simulink model "Demo_MinDef_Aug2013"  (Simulink 7.7)
settings: Solver=ode4  StartTime=0.0  StopTime=inf  FixedStep=sample_time_Vicon  RelTol=1e-3
InitFcn:
  | sample_time_Vicon = 0.005;
  | sample_time=0.02;
  | DeltaT = sample_time;
  | H0 = 0.35;
  | Kl = 1;
  | Omega_r =1.2; %1.2
  | Omega_c = 1.2;
  | omega_circle = 36*pi/180;
  | omega_h = 0.1;%Ascending speed
  | PI = pi;
undefined symbols (not defined in the file or in its folder): DiscIntNeverNeededParam
libraries: simulink x22, dspadpt3 x8
(part 4 of 4)

== system Demo_MinDef_Aug2013/Vicon_Data/Raw Quad Pose from Vicon/Process Vicon Raw Data1/Flip_pi1/Flip_0_to_2pi/Flip_2pi ==
  Angle : Inport
  Bias : Bias  Bias=-2*pi
  Constant : Constant  Value=2*pi
  Data Type Duplicate : DataTypeDuplicate
  Modulo : Math  Operator=mod  SaturateOnIntegerOverflow=on
  Sign1 : Signum
  Switch : Switch
  Angle_Flip : Outport
  wires:
  Angle/1 -> Modulo/1, Sign1/1, Data Type Duplicate/1
  Constant/1 -> Modulo/2
  Modulo/1 -> Bias/1, Switch/1
  Sign1/1 -> Switch/2
  Bias/1 -> Switch/3
  Switch/1 -> Angle_Flip/1, Data Type Duplicate/2

== system Demo_MinDef_Aug2013/Vicon_Data/Raw Quad Pose from Vicon/Process Vicon Raw Data2/Flip_pi1/Flip_0_to_2pi/Flip_2pi ==
  Angle : Inport
  Bias : Bias  Bias=-2*pi
  Constant : Constant  Value=2*pi
  Data Type Duplicate : DataTypeDuplicate
  Modulo : Math  Operator=mod  SaturateOnIntegerOverflow=on
  Sign1 : Signum
  Switch : Switch
  Angle_Flip : Outport
  wires:
  Switch/1 -> Data Type Duplicate/2, Angle_Flip/1
  Bias/1 -> Switch/3
  Sign1/1 -> Switch/2
  Modulo/1 -> Switch/1, Bias/1
  Constant/1 -> Modulo/2
  Angle/1 -> Data Type Duplicate/1, Sign1/1, Modulo/1

== system Demo_MinDef_Aug2013/Vicon_Data/Raw Quad Pose from Vicon/Process Vicon Raw Data3/Flip_pi1/Flip_0_to_2pi/Flip_2pi ==
  Angle : Inport
  Bias : Bias  Bias=-2*pi
  Constant : Constant  Value=2*pi
  Data Type Duplicate : DataTypeDuplicate
  Modulo : Math  Operator=mod  SaturateOnIntegerOverflow=on
  Sign1 : Signum
  Switch : Switch
  Angle_Flip : Outport
  wires:
  Angle/1 -> Modulo/1, Sign1/1, Data Type Duplicate/1
  Constant/1 -> Modulo/2
  Modulo/1 -> Bias/1, Switch/1
  Sign1/1 -> Switch/2
  Bias/1 -> Switch/3
  Switch/1 -> Angle_Flip/1, Data Type Duplicate/2

== system Demo_MinDef_Aug2013/Vicon_Data/Raw Quad Pose from Vicon/Process Vicon Raw Data4/Flip_pi1/Flip_0_to_2pi/Flip_2pi ==
  Angle : Inport
  Bias : Bias  Bias=-2*pi
  Constant : Constant  Value=2*pi
  Data Type Duplicate : DataTypeDuplicate
  Modulo : Math  Operator=mod  SaturateOnIntegerOverflow=on
  Sign1 : Signum
  Switch : Switch
  Angle_Flip : Outport
  wires:
  Switch/1 -> Data Type Duplicate/2, Angle_Flip/1
  Bias/1 -> Switch/3
  Sign1/1 -> Switch/2
  Modulo/1 -> Switch/1, Bias/1
  Constant/1 -> Modulo/2
  Angle/1 -> Data Type Duplicate/1, Sign1/1, Modulo/1

== system Demo_MinDef_Aug2013/Vicon_Data/Raw Quad Pose from Vicon/Process Vicon Raw Data5/Flip_pi1/Flip_0_to_2pi/Flip_2pi ==
  Angle : Inport
  Bias : Bias  Bias=-2*pi
  Constant : Constant  Value=2*pi
  Data Type Duplicate : DataTypeDuplicate
  Modulo : Math  Operator=mod  SaturateOnIntegerOverflow=on
  Sign1 : Signum
  Switch : Switch
  Angle_Flip : Outport
  wires:
  Switch/1 -> Data Type Duplicate/2, Angle_Flip/1
  Bias/1 -> Switch/3
  Sign1/1 -> Switch/2
  Modulo/1 -> Switch/1, Bias/1
  Constant/1 -> Modulo/2
  Angle/1 -> Data Type Duplicate/1, Sign1/1, Modulo/1

== system Demo_MinDef_Aug2013/Vicon_Data/Raw Quad Pose from Vicon/Process Vicon Raw Data6/Flip_pi1/Flip_0_to_2pi/Flip_2pi ==
  Angle : Inport
  Bias : Bias  Bias=-2*pi
  Constant : Constant  Value=2*pi
  Data Type Duplicate : DataTypeDuplicate
  Modulo : Math  Operator=mod  SaturateOnIntegerOverflow=on
  Sign1 : Signum
  Switch : Switch
  Angle_Flip : Outport
  wires:
  Angle/1 -> Modulo/1, Sign1/1, Data Type Duplicate/1
  Constant/1 -> Modulo/2
  Modulo/1 -> Bias/1, Switch/1
  Sign1/1 -> Switch/2
  Bias/1 -> Switch/3
  Switch/1 -> Angle_Flip/1, Data Type Duplicate/2

== system Demo_MinDef_Aug2013/Vicon_Data/Raw Quad Pose from Vicon/Process Vicon Raw Data7/Flip_pi1/Flip_0_to_2pi/Flip_2pi ==
  Angle : Inport
  Bias : Bias  Bias=-2*pi
  Constant : Constant  Value=2*pi
  Data Type Duplicate : DataTypeDuplicate
  Modulo : Math  Operator=mod  SaturateOnIntegerOverflow=on
  Sign1 : Signum
  Switch : Switch
  Angle_Flip : Outport
  wires:
  Switch/1 -> Data Type Duplicate/2, Angle_Flip/1
  Bias/1 -> Switch/3
  Sign1/1 -> Switch/2
  Modulo/1 -> Switch/1, Bias/1
  Constant/1 -> Modulo/2
  Angle/1 -> Data Type Duplicate/1, Sign1/1, Modulo/1

== system Demo_MinDef_Aug2013/Vicon_Data/Raw Quad Pose from Vicon/Process Vicon Raw Data8/Flip_pi1/Flip_0_to_2pi/Flip_2pi ==
  Angle : Inport
  Bias : Bias  Bias=-2*pi
  Constant : Constant  Value=2*pi
  Data Type Duplicate : DataTypeDuplicate
  Modulo : Math  Operator=mod  SaturateOnIntegerOverflow=on
  Sign1 : Signum
  Switch : Switch
  Angle_Flip : Outport
  wires:
  Angle/1 -> Modulo/1, Sign1/1, Data Type Duplicate/1
  Constant/1 -> Modulo/2
  Modulo/1 -> Bias/1, Switch/1
  Sign1/1 -> Switch/2
  Bias/1 -> Switch/3
  Switch/1 -> Angle_Flip/1, Data Type Duplicate/2

== stateflow chart Quad 5 Planning/Trajectory Logic/UAV SF1 ==
  state Landing
    state Decsending
      en:PosDesired = Pos;
      du:PosDesired[2] = (0 - PosDesired[2])*1*DeltaT + PosDesired[2] ;
    state CutThrottle
      du:HoverThrottle = (0.01 - HoverThrottle)*2*DeltaT + HoverThrottle ;
    (default) -> Decsending
    Decsending -> CutThrottle : [Pos[2] > -0.15]
  state Airborne
    state TakeOff
      du:HoverThrottle = (H0 - HoverThrottle)*2*DeltaT + HoverThrottle ;
    state Hover
      en: PosDesired[2] = -1;
    state Trajectory
      state SpiralAscend
        du: PosDesired[0] = 2*sin(0.0 + T_circle*omega_circle);
        PosDesired[1] = 2*cos(0.0 + T_circle*omega_circle);
        PosDesired[2] = max(-2,-1 - T_circle*omega_h);
        T_circle = T_circle + DeltaT;
      state Circle2D
        du: PosDesired[0] = 2*sin(150*PI/180 + T_circle*omega_circle);
        PosDesired[1] = 2*cos(150*PI/180 + T_circle*omega_circle);
        T_circle = T_circle + DeltaT;
      state SpiralDescend
        du: PosDesired[0] = 2*sin((720- 180/2)*PI/180 + T_circle*omega_circle);
        PosDesired[1] = 2*cos((720- 180/2)*PI/180 + T_circle*omega_circle);
        PosDesired[2] =min(-1,-2 + T_circle*omega_h);
        T_circle = T_circle + DeltaT;
      state Hex1
        en: PosDesired[0] = 1.5*sin(150*PI/180);
        PosDesired[1] = 1.5*cos(150*PI/180);
        PosDesired[2] = -1;
      state Line2
        en: PosDesired[0] = -1; PosDesired[1] =-1; PosDesired[2] = -1;
      state Line1
        en: PosDesired[0] = 0; PosDesired[1] = -1; PosDesired[2] = -1;
      state Line3
        en: PosDesired[0] = 1; PosDesired[1] =-1; PosDesired[2] = -2;
      state Hex
        en: PosDesired[0] = 1.5*sin(150*PI/180); PosDesired[1] = 1.5*cos(150*PI/180);
      state Line4
        en: PosDesired[0] = 0; PosDesired[1] = -1; PosDesired[2] = -1;
      Circle2D -> SpiralAscend : [T_circle*omega_circle*180/PI > (390 +180)]
          | {T_circle =0.0;}
      SpiralAscend -> SpiralDescend : [T_circle*omega_circle *180/PI > (720-180/2)]
          | {T_circle =0.0;}
      SpiralDescend -> Hex1 : [T_circle*omega_circle *180/PI > (720-180/2)]
          | {T_circle =0.0;}
      (default) -> Line1 : {line_count = -1;}
      Line1 -> Line2 : after (10, sec)
      Line2 -> Line3 : after (5, sec)
      Line3 -> Line4 : after (5, sec)
      Hex -> Circle2D : after (10, sec)
          | {T_circle = 0.0;}
      Line4 -> Hex : after (5, sec)
    (default) -> TakeOff : {PosDesired = Pos;  PosDesired[2] = -1;}
    TakeOff -> Hover : after(5,sec)
        | {PosDesired = Pos;}
    Hover -> Trajectory : [RC[5] > 0]
    Trajectory -> Hover : [RC[5] < 0]
        | {PosDesired = Pos;}
  (default) -> Landing : {HoverThrottle=0.01;}
  Airborne -> Landing : [RC[6] < -0.5]
  Landing -> Airborne : [RC[6] > 0.5]
  data: PosDesired output double size=4; HoverThrottle output double size=1; Mode output uint8 size=3; RC input double size=8; Pos input double size=4; PerchPos input double size=4; DeltaT parameter double size=1; H0 parameter double size=1; Kl parameter double size=1; VelCmd local double size=2 =0; line_count local int8 size=1 =0; triangle_count local int8 size=1 =0; T_circle local double size=1; omega_circle parameter double size=1; PI parameter double size=1; omega_h parameter double size=1

== stateflow chart Quad 1 Planning/Trajectory Logic/UAV SF1 ==
  state Landing
    state Decsending
      en:PosDesired = Pos;
      du:PosDesired[2] = (0 - PosDesired[2])*1*DeltaT + PosDesired[2] ;
    state CutThrottle
      du:HoverThrottle = (0.01 - HoverThrottle)*2*DeltaT + HoverThrottle ;
    (default) -> Decsending
    Decsending -> CutThrottle : [Pos[2] > -0.15]
  state Airborne
    state TakeOff
      du:HoverThrottle = (H0 - HoverThrottle)*2*DeltaT + HoverThrottle ;
    state Hover
      en: PosDesired[2] = -1;
    state Trajectory
      state SpiralDescend
        du: PosDesired[0] = 2*sin( (720- 300/2)*PI/180 + T_circle*omega_circle);
        PosDesired[1] = 2*cos((720- 300/2)*PI/180 + T_circle*omega_circle);
        PosDesired[2] =min(-1,-2 + T_circle*omega_h);
        T_circle = T_circle + DeltaT;
      state Hex1
        en: PosDesired[0] = 1.5*sin(30*PI/180);
        PosDesired[1] = 1.5*cos(30*PI/180);
        PosDesired[2] = -1;
      state SpiralAscend
        du: PosDesired[0] = 2*sin(0.0 + T_circle*omega_circle);
        PosDesired[1] = 2*cos(0.0 + T_circle*omega_circle);
        PosDesired[2] = max(-2,-1 - T_circle*omega_h);
        T_circle = T_circle + DeltaT;
      state Circle2D
        du: PosDesired[0] = 2*sin(30*PI/180 + T_circle*omega_circle);
        PosDesired[1] = 2*cos(30*PI/180 + T_circle*omega_circle);
        T_circle = T_circle + DeltaT;
      state Line2
        en: PosDesired[0] = -1; PosDesired[1] = 2.6; PosDesired[2] = -1;
      state Line1
        en: PosDesired[0] = 0; PosDesired[1] = 2.6; PosDesired[2] = -1;
      state Line3
        en: PosDesired[0] = 1; PosDesired[1] = 2.6; PosDesired[2] = -2;
      state Hex
        en: PosDesired[0] = 1.5*sin(30*PI/180); PosDesired[1] = 1.5*cos(30*PI/180);
      state Line4
        en: PosDesired[0] = 0; PosDesired[1] = 2.6; PosDesired[2] = -1;
      SpiralDescend -> Hex1 : [T_circle*omega_circle *180/PI > (720- 300/2)]
          | {T_circle =0.0;}
      SpiralAscend -> SpiralDescend : [T_circle*omega_circle *180/PI > (720- 300/2)]
          | {T_circle =0.0;}
      Circle2D -> SpiralAscend : [T_circle*omega_circle*180/PI > (390 +300)]
          | {T_circle =0.0;}
      (default) -> Line1 : {line_count = -1;}
      Line1 -> Line2 : after (10, sec)
      Line2 -> Line3 : after (5, sec)
      Line3 -> Line4 : after (5, sec)
      Hex -> Circle2D : after (10, sec)
          | {T_circle = 0.0;}
      Line4 -> Hex : after (5, sec)
    (default) -> TakeOff : {PosDesired = Pos;  PosDesired[2] = -1;}
    TakeOff -> Hover : after(5,sec)
        | {PosDesired = Pos;}
    Hover -> Trajectory : [RC[5] > 0]
    Trajectory -> Hover : [RC[5] < 0]
        | {PosDesired = Pos;}
  (default) -> Landing : {HoverThrottle=0.01;}
  Airborne -> Landing : [RC[6] < -0.5]
  Landing -> Airborne : [RC[6] > 0.5]
  data: PosDesired output double size=4; HoverThrottle output double size=1; Mode output uint8 size=3; RC input double size=8; Pos input double size=4; PerchPos input double size=4; DeltaT parameter double size=1; H0 parameter double size=1; Kl parameter double size=1; VelCmd local double size=2 =0; line_count local int8 size=1 =0; triangle_count local int8 size=1 =0; T_circle local double size=1; omega_circle parameter double size=1; PI parameter double size=1; omega_h parameter double

== stateflow chart Quad 4 Planning/Trajectory Logic/UAV SF1 ==
  state Landing
    state Decsending
      en:PosDesired = Pos;
      du:PosDesired[2] = (0 - PosDesired[2])*1*DeltaT + PosDesired[2] ;
    state CutThrottle
      du:HoverThrottle = (0.01 - HoverThrottle)*2*DeltaT + HoverThrottle ;
    (default) -> Decsending
    Decsending -> CutThrottle : [Pos[2] > -0.15]
  state Airborne
    state TakeOff
      du:HoverThrottle = (H0 - HoverThrottle)*2*DeltaT + HoverThrottle ;
    state Hover
      en: PosDesired[2] = -1;
    state Trajectory
      state SpiralAscend
        du: PosDesired[0] = 2*sin(0.0 + T_circle*omega_circle);
        PosDesired[1] = 2*cos(0.0 + T_circle*omega_circle);
        PosDesired[2] = max(-2,-1 - T_circle*omega_h);
        T_circle = T_circle + DeltaT;
      state Circle2D
        du: PosDesired[0] = 2*sin(270*PI/180 + T_circle*omega_circle);
        PosDesired[1] = 2*cos(270*PI/180 + T_circle*omega_circle);
        T_circle = T_circle + DeltaT;
      state SpiralDescend
        du: PosDesired[0] = 2*sin((720- 60/2)*PI/180 + T_circle*omega_circle);
        PosDesired[1] = 2*cos((720- 60/2)*PI/180 + T_circle*omega_circle);
        PosDesired[2] =min(-1,-2 + T_circle*omega_h);
        T_circle = T_circle + DeltaT;
      state Hex1
        en: PosDesired[0] = 1.5*sin(270*PI/180);
        PosDesired[1] = 1.5*cos(270*PI/180);
        PosDesired[2] = -1;
      state Line2
        en: PosDesired[0] = -1; PosDesired[1] =0; PosDesired[2] = -1;
      state Line1
        en: PosDesired[0] = 0; PosDesired[1] = 0; PosDesired[2] = -1;
      state Line3
        en: PosDesired[0] = 1; PosDesired[1] =0; PosDesired[2] = -1;
      state Hex
        en: PosDesired[0] = 1.5*sin(270*PI/180); PosDesired[1] = 1.5*cos(270*PI/180);
      state Line4
        en: PosDesired[0] = 0; PosDesired[1] = 0; PosDesired[2] = -1;
      Circle2D -> SpiralAscend : [T_circle*omega_circle*180/PI > (390 +60)]
          | {T_circle =0.0;}
      SpiralAscend -> SpiralDescend : [T_circle*omega_circle *180/PI > (720-60/2)]
          | {T_circle =0.0;}
      SpiralDescend -> Hex1 : [T_circle*omega_circle *180/PI > (720-60/2)]
          | {T_circle =0.0;}
      (default) -> Line1 : {line_count = -1;}
      Line1 -> Line2 : after (10, sec)
      Line2 -> Line3 : after (5, sec)
      Line3 -> Line4 : after (5, sec)
      Hex -> Circle2D : after (10, sec)
          | {T_circle = 0.0;}
      Line4 -> Hex : after (5, sec)
    (default) -> TakeOff : {PosDesired = Pos;  PosDesired[2] = -1;}
    TakeOff -> Hover : after(5,sec)
        | {PosDesired = Pos;}
    Hover -> Trajectory : [RC[5] > 0]
    Trajectory -> Hover : [RC[5] < 0]
        | {PosDesired = Pos;}
  (default) -> Landing : {HoverThrottle=0.01;}
  Airborne -> Landing : [RC[6] < -0.5]
  Landing -> Airborne : [RC[6] > 0.5]
  data: PosDesired output double size=4; HoverThrottle output double size=1; Mode output uint8 size=3; RC input double size=8; Pos input double size=4; PerchPos input double size=4; DeltaT parameter double size=1; H0 parameter double size=1; Kl parameter double size=1; VelCmd local double size=2 =0; line_count local int8 size=1 =0; triangle_count local int8 size=1 =0; T_circle local double size=1; omega_circle parameter double size=1; PI parameter double size=1; omega_h parameter double size=1

== matlab function Quad 2 Planning/Yaw Controller/MATLAB Function ==
  data: u input double; y output double
function y = fcn(u)
%#codegen
y = u;
if y > pi    
    y = y - 2*pi;
elseif y < -pi
        y = y + 2*pi;
end

== stateflow chart Quad 3 Planning/Trajectory Logic/UAV SF1 ==
  state Landing
    state Decsending
      en:PosDesired = Pos;
      du:PosDesired[2] = (0 - PosDesired[2])*1*DeltaT + PosDesired[2] ;
    state CutThrottle
      du:HoverThrottle = (0.01 - HoverThrottle)*2*DeltaT + HoverThrottle ;
    (default) -> Decsending
    Decsending -> CutThrottle : [Pos[2] > -0.15]
  state Airborne
    state TakeOff
      du:HoverThrottle = (H0 - HoverThrottle)*2*DeltaT + HoverThrottle ;
    state Hover
      en: PosDesired[2] = -1;
    state Trajectory
      state SpiralAscend
        du: PosDesired[0] = 2*sin(0.0 + T_circle*omega_circle);
        PosDesired[1] = 2*cos(0.0 + T_circle*omega_circle);
        PosDesired[2] =max( -2,-1 - T_circle*omega_h);
        T_circle = T_circle + DeltaT;
      state Circle2D
        du: PosDesired[0] = 2*sin(90*PI/180 + T_circle*omega_circle);
        PosDesired[1] = 2*cos(90*PI/180 + T_circle*omega_circle);
        T_circle = T_circle + DeltaT;
      state SpiralDescend
        du: PosDesired[0] = 2*sin((720- 240/2)*PI/180 + T_circle*omega_circle);
        PosDesired[1] = 2*cos((720- 240/2)*PI/180 + T_circle*omega_circle);
        PosDesired[2] =min(-1,-2 + T_circle*omega_h);
        T_circle = T_circle + DeltaT;
      state Hex1
        en: PosDesired[0] = 1.5*sin(90*PI/180);
        PosDesired[1] = 1.5*cos(90*PI/180);
        PosDesired[2] = -1;
      state Line2
        en: PosDesired[0] = -1; PosDesired[1] = 1; PosDesired[2] = -1;
      state Line1
        en: PosDesired[0] = 0; PosDesired[1] = 1; PosDesired[2] = -1;
      state Line3
        en: PosDesired[0] = 1; PosDesired[1] = 1; PosDesired[2] = -2;
      state Hex
        en: PosDesired[0] = 1.5*sin(90*PI/180); PosDesired[1] = 1.5*cos(90*PI/180);
      state Line4
        en: PosDesired[0] = 0; PosDesired[1] = 1; PosDesired[2] = -1;
      Circle2D -> SpiralAscend : [T_circle*omega_circle*180/PI > (390 +240)]
          | {T_circle =0.0;}
      SpiralAscend -> SpiralDescend : [T_circle*omega_circle *180/PI > (720-240/2)]
          | {T_circle =0.0;}
      SpiralDescend -> Hex1 : [T_circle*omega_circle *180/PI > (720-240/2)]
          | {T_circle =0.0;}
      (default) -> Line1 : {line_count = -1;}
      Line1 -> Line2 : after (10, sec)
      Line2 -> Line3 : after (5, sec)
      Line3 -> Line4 : after (5, sec)
      Hex -> Circle2D : after (10, sec)
          | {T_circle = 0.0;}
      Line4 -> Hex : after (5, sec)
    (default) -> TakeOff : {PosDesired = Pos;  PosDesired[2] = -1;}
    TakeOff -> Hover : after(5,sec)
        | {PosDesired = Pos;}
    Hover -> Trajectory : [RC[5] > 0]
    Trajectory -> Hover : [RC[5] < 0]
        | {PosDesired = Pos;}
  (default) -> Landing : {HoverThrottle=0.01;}
  Airborne -> Landing : [RC[6] < -0.5]
  Landing -> Airborne : [RC[6] > 0.5]
  data: PosDesired output double size=4; HoverThrottle output double size=1; Mode output uint8 size=3; RC input double size=8; Pos input double size=4; PerchPos input double size=4; DeltaT parameter double size=1; H0 parameter double size=1; Kl parameter double size=1; VelCmd local double size=2 =0; line_count local int8 size=1 =0; triangle_count local int8 size=1 =0; T_circle local double size=1; omega_circle parameter double size=1; PI parameter double size=1; omega_h parameter double size=1

== matlab function Quad 4 Planning/Yaw Controller/MATLAB Function ==
  data: u input double; y output double
function y = fcn(u)
%#codegen
y = u;
if y > pi    
    y = y - 2*pi;
elseif y < -pi
        y = y + 2*pi;
end

== stateflow chart Quad 2 Planning/Trajectory Logic/UAV SF1 ==
  state Landing
    state Decsending
      en:PosDesired = Pos;
      du:PosDesired[2] = (0 - PosDesired[2])*1*DeltaT + PosDesired[2] ;
    state CutThrottle
      du:HoverThrottle = (0.01 - HoverThrottle)*2*DeltaT + HoverThrottle ;
    (default) -> Decsending
    Decsending -> CutThrottle : [Pos[2] > -0.15]
  state Airborne
    state TakeOff
      du:HoverThrottle = (H0 - HoverThrottle)*2*DeltaT + HoverThrottle ;
    state Hover
      en: PosDesired[2] = -1;
    state Trajectory
      state Line1
        en: PosDesired[0] = 0; PosDesired[1] = 1.8; PosDesired[2] = -1;
      state Line4
        en: PosDesired[0] = 0; PosDesired[1] = 1.8; PosDesired[2] = -1;
      state Hex
        en: PosDesired[0] = 1.5*sin(330*PI/180); PosDesired[1] = 1.5*cos(330*PI/180);
      state Circle2D
        du: PosDesired[0] = 2*sin(330*PI/180 + T_circle*omega_circle);
        PosDesired[1] = 2*cos(330*PI/180 + T_circle*omega_circle);
        T_circle = T_circle + DeltaT;
      state SpiralAscend
        du: PosDesired[0] = 2*sin(0.0 + T_circle*omega_circle);
        PosDesired[1] = 2*cos(0.0 + T_circle*omega_circle);
        PosDesired[2] = max(-2,-1 - T_circle*omega_h);
        T_circle = T_circle + DeltaT;
      state SpiralDescend
        du: PosDesired[0] = 2*sin(0.0 + T_circle*omega_circle);
        PosDesired[1] = 2*cos(0.0 + T_circle*omega_circle);
        PosDesired[2] =min(-1,-2 + T_circle*omega_h);
        T_circle = T_circle + DeltaT;
      state Hex1
        en: PosDesired[0] = 1.5*sin(330*PI/180);
        PosDesired[1] = 1.5*cos(330*PI/180);
        PosDesired[2] = -1;
      state Line2
        en: PosDesired[0] = -1; PosDesired[1] = 1.8; PosDesired[2] = -1;
      state Line3
        en: PosDesired[0] = 1; PosDesired[1] = 1.8; PosDesired[2] = -1;
      (default) -> Line1 : {line_count = -1;}
      Line1 -> Line2 : after (10, sec)
      Hex -> Circle2D : after (10, sec)
          | {T_circle = 0.0;}
      Circle2D -> SpiralAscend : [T_circle*omega_circle*180/PI > 390]
          | {T_circle =0.0;}
      SpiralAscend -> SpiralDescend : [T_circle*omega_circle *180/PI > 720]
          | {T_circle =0.0;}
      SpiralDescend -> Hex1 : [T_circle*omega_circle *180/PI > 720]
          | {T_circle =0.0;}
      Line4 -> Hex : after (5, sec)
      Line2 -> Line3 : after (5, sec)
      Line3 -> Line4 : after (5, sec)
    (default) -> TakeOff : {PosDesired = Pos;  PosDesired[2] = -1;}
    TakeOff -> Hover : after(5,sec)
        | {PosDesired = Pos;}
    Hover -> Trajectory : [RC[5] > 0]
    Trajectory -> Hover : [RC[5] < 0]
        | {PosDesired = Pos;}
  (default) -> Landing : {HoverThrottle=0.01;}
  Airborne -> Landing : [RC[6] < -0.5]
  Landing -> Airborne : [RC[6] > 0.5]
  data: PosDesired output double size=4; HoverThrottle output double size=1; Mode output uint8 size=3; RC input double size=8; Pos input double size=4; PerchPos input double size=4; DeltaT parameter double size=1; H0 parameter double size=1; Kl parameter double size=1; VelCmd local double size=2 =0; line_count local int8 size=1 =0; triangle_count local int8 size=1 =0; T_circle local double size=1; omega_circle parameter double size=1; PI parameter double size=1; omega_h parameter double size=1

== matlab function Quad 3 Planning/Yaw Controller/MATLAB Function ==
  data: u input double; y output double
function y = fcn(u)
%#codegen
y = u;
if y > pi    
    y = y - 2*pi;
elseif y < -pi
        y = y + 2*pi;
end

== matlab function Quad 1 Planning/Yaw Controller/MATLAB Function ==
  data: u input double; y output double
function y = fcn(u)
%#codegen
y = u;
if y > pi    
    y = y - 2*pi;
elseif y < -pi
        y = y + 2*pi;
end

== matlab function Quad 5 Planning/Yaw Controller/MATLAB Function ==
  data: u input double; y output double
function y = fcn(u)
%#codegen
y = u;
if y > pi    
    y = y - 2*pi;
elseif y < -pi
        y = y + 2*pi;
end

== stateflow chart Quad 6 Planning /Trajectory Logic/UAV SF ==
  state Landing
    state Decsending
      en:PosDesired = Pos;
      du:PosDesired[2] = (0 - PosDesired[2])*1*DeltaT + PosDesired[2] ;
    state CutThrottle
      du:HoverThrottle = (0.01 - HoverThrottle)*2*DeltaT + HoverThrottle ;
    (default) -> Decsending
    Decsending -> CutThrottle : [Pos[2] > -0.15]
  state Airborne
    state TakeOff
      du:HoverThrottle = (H0 - HoverThrottle)*2*DeltaT + HoverThrottle ;
    state Hover
      en: PosDesired[2] = -1;
    state Trajectory
      state SpiralAscend
        du: PosDesired[0] = 2*sin(0.0 + T_circle*omega_circle);
        PosDesired[1] = 2*cos(0.0 + T_circle*omega_circle);
        PosDesired[2] = max(-2,-1 - T_circle*omega_h);
        T_circle = T_circle + DeltaT;
      state Circle2D
        du: PosDesired[0] = 2*sin(210*PI/180 + T_circle*omega_circle);
        PosDesired[1] = 2*cos(210*PI/180 + T_circle*omega_circle);
        T_circle = T_circle + DeltaT;
      state SpiralDescend
        du: PosDesired[0] = 2*sin( (720-120/2)*PI/180 + T_circle*omega_circle);
        PosDesired[1] = 2*cos((720-120/2)*PI/180 + T_circle*omega_circle);
        PosDesired[2] =min(-1,-2 + T_circle*omega_h);
        T_circle = T_circle + DeltaT;
      state Hex1
        en: PosDesired[0] = 1.5*sin(210*PI/180);
        PosDesired[1] = 1.5*cos(210*PI/180);
        PosDesired[2] = -1;
      state Line2
        en: PosDesired[0] = -1; PosDesired[1] = -2; PosDesired[2] = -1;
      state Line1
        en: PosDesired[0] = 0; PosDesired[1] = -2; PosDesired[2] = -1;
      state Line3
        en: PosDesired[0] = 1; PosDesired[1] = -2; PosDesired[2] = -1;
      state Hex
        en: PosDesired[0] = 1.5*sin(210*PI/180); PosDesired[1] = 1.5*cos(210*PI/180);
      state Line4
        en: PosDesired[0] = 0; PosDesired[1] = -2; PosDesired[2] = -1;
      Circle2D -> SpiralAscend : [T_circle*omega_circle*180/PI > (390 +120)]
          | {T_circle =0.0;}
      SpiralAscend -> SpiralDescend : [T_circle*omega_circle *180/PI > (720-120/2)]
          | {T_circle =0.0;}
      SpiralDescend -> Hex1 : [T_circle*omega_circle *180/PI > (720-120/2)]
          | {T_circle =0.0;}
      (default) -> Line1 : {line_count = -1;}
      Line1 -> Line2 : after (10, sec)
      Line2 -> Line3 : after (5, sec)
      Line3 -> Line4 : after (5, sec)
      Hex -> Circle2D : after (10, sec)
          | {T_circle = 0.0;}
      Line4 -> Hex : after (5, sec)
    (default) -> TakeOff : {PosDesired = Pos;  PosDesired[2] = -1;}
    TakeOff -> Hover : after(5,sec)
        | {PosDesired = Pos;}
    Hover -> Trajectory : [RC[5] > 0]
    Trajectory -> Hover : [RC[5] < 0]
        | {PosDesired = Pos;}
  (default) -> Landing : {HoverThrottle=0.01;}
  Airborne -> Landing : [RC[6] < -0.5]
  Landing -> Airborne : [RC[6] > 0.5]
  data: PosDesired output double size=4; HoverThrottle output double size=1; Mode output uint8 size=3; RC input double size=8; Pos input double size=4; PerchPos input double size=4; DeltaT parameter double size=1; H0 parameter double size=1; Kl parameter double size=1; VelCmd local double size=2 =0; line_count local int8 size=1 =0; triangle_count local int8 size=1 =0; T_circle local double size=1; omega_circle parameter double size=1; PI parameter double size=1; omega_h parameter double size=1

== matlab function Quad 6 Planning /Yaw Controller/MATLAB Function ==
  data: u input double; y output double
function y = fcn(u)
%#codegen
y = u;
if y > pi    
    y = y - 2*pi;
elseif y < -pi
        y = y + 2*pi;
end
